simulink model "Microstick_II_33EP128MC202_Drotek_I2C_MS5611_TempAndPressure"  (Simulink 7.5)
settings: Solver=FixedStepDiscrete  StartTime=0.0  StopTime=10.0  FixedStep=0.01  RelTol=1e-3
undefined symbols (not defined in the file or in its folder): A0, A4, B10, B11, B8, B9, magnitude, Max, ms, P20, P42, P43, Pin, Resol, Slope1, Slope2, us
libraries: simulink x30, MCHP_Blockset x16
(part 2 of 2)

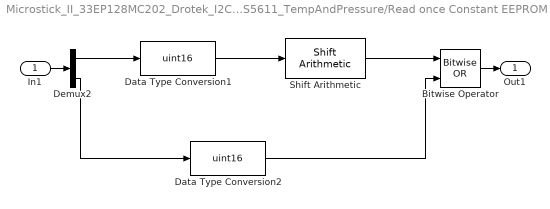
== system Microstick_II_33EP128MC202_Drotek_I2C_MS5611_TempAndPressure/Read once Constant EEPROM Calibration data From MS5611 (Blocking I2C blocks)/  ==
  In1 : Inport
  Bitwise Operator : simulink/Logic and Bit Operations/Bitwise Operator  logicop=OR  UseBitMask=off  NumInputPorts=2  BitMask=bin2dec('11011001')  BitMaskRealWorld=Stored Integer
  Data Type Conversion1 : DataTypeConversion  OutDataTypeMode=uint16  OutDataTypeStr=uint16
  Data Type Conversion2 : DataTypeConversion  OutDataTypeMode=uint16  OutDataTypeStr=uint16
  Demux2 : Demux  Outputs=2
  Shift Arithmetic : simulink/Logic and Bit Operations/Shift Arithmetic  SystemSampleTime=-1  nBitShiftRight=-8  nBinPtShiftRight=0
  Out1 : Outport
  wires:
  In1/1 -> Demux2/1
  Bitwise Operator/1 -> Out1/1
  Data Type Conversion1/1 -> Shift Arithmetic/1
  Demux2/2 -> Data Type Conversion2/1
  Shift Arithmetic/1 -> Bitwise Operator/1
  Demux2/1 -> Data Type Conversion1/1
  Data Type Conversion2/1 -> Bitwise Operator/2

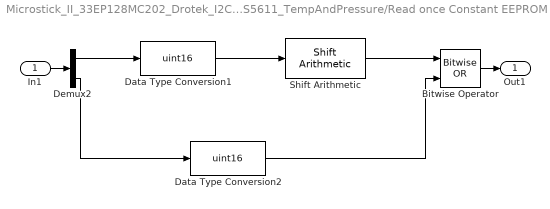
== system Microstick_II_33EP128MC202_Drotek_I2C_MS5611_TempAndPressure/Read once Constant EEPROM Calibration data From MS5611 (Blocking I2C blocks)/ 1 ==
  In1 : Inport
  Bitwise Operator : simulink/Logic and Bit Operations/Bitwise Operator  logicop=OR  UseBitMask=off  NumInputPorts=2  BitMask=bin2dec('11011001')  BitMaskRealWorld=Stored Integer
  Data Type Conversion1 : DataTypeConversion  OutDataTypeMode=uint16  OutDataTypeStr=uint16
  Data Type Conversion2 : DataTypeConversion  OutDataTypeMode=uint16  OutDataTypeStr=uint16
  Demux2 : Demux  Outputs=2
  Shift Arithmetic : simulink/Logic and Bit Operations/Shift Arithmetic  SystemSampleTime=-1  nBitShiftRight=-8  nBinPtShiftRight=0
  Out1 : Outport
  wires:
  Data Type Conversion2/1 -> Bitwise Operator/2
  Demux2/1 -> Data Type Conversion1/1
  Shift Arithmetic/1 -> Bitwise Operator/1
  Demux2/2 -> Data Type Conversion2/1
  Data Type Conversion1/1 -> Shift Arithmetic/1
  Bitwise Operator/1 -> Out1/1
  In1/1 -> Demux2/1

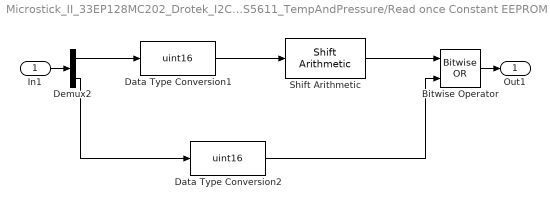
== system Microstick_II_33EP128MC202_Drotek_I2C_MS5611_TempAndPressure/Read once Constant EEPROM Calibration data From MS5611 (Blocking I2C blocks)/ 2 ==
  In1 : Inport
  Bitwise Operator : simulink/Logic and Bit Operations/Bitwise Operator  logicop=OR  UseBitMask=off  NumInputPorts=2  BitMask=bin2dec('11011001')  BitMaskRealWorld=Stored Integer
  Data Type Conversion1 : DataTypeConversion  OutDataTypeMode=uint16  OutDataTypeStr=uint16
  Data Type Conversion2 : DataTypeConversion  OutDataTypeMode=uint16  OutDataTypeStr=uint16
  Demux2 : Demux  Outputs=2
  Shift Arithmetic : simulink/Logic and Bit Operations/Shift Arithmetic  SystemSampleTime=-1  nBitShiftRight=-8  nBinPtShiftRight=0
  Out1 : Outport
  wires:
  In1/1 -> Demux2/1
  Bitwise Operator/1 -> Out1/1
  Data Type Conversion1/1 -> Shift Arithmetic/1
  Demux2/2 -> Data Type Conversion2/1
  Shift Arithmetic/1 -> Bitwise Operator/1
  Demux2/1 -> Data Type Conversion1/1
  Data Type Conversion2/1 -> Bitwise Operator/2

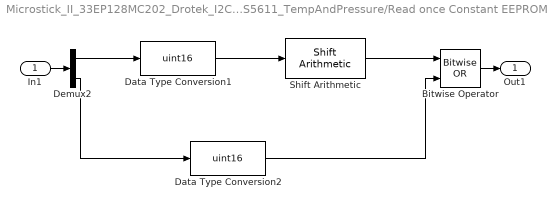
== system Microstick_II_33EP128MC202_Drotek_I2C_MS5611_TempAndPressure/Read once Constant EEPROM Calibration data From MS5611 (Blocking I2C blocks)/ 3 ==
  In1 : Inport
  Bitwise Operator : simulink/Logic and Bit Operations/Bitwise Operator  logicop=OR  UseBitMask=off  NumInputPorts=2  BitMask=bin2dec('11011001')  BitMaskRealWorld=Stored Integer
  Data Type Conversion1 : DataTypeConversion  OutDataTypeMode=uint16  OutDataTypeStr=uint16
  Data Type Conversion2 : DataTypeConversion  OutDataTypeMode=uint16  OutDataTypeStr=uint16
  Demux2 : Demux  Outputs=2
  Shift Arithmetic : simulink/Logic and Bit Operations/Shift Arithmetic  SystemSampleTime=-1  nBitShiftRight=-8  nBinPtShiftRight=0
  Out1 : Outport
  wires:
  Data Type Conversion2/1 -> Bitwise Operator/2
  Demux2/1 -> Data Type Conversion1/1
  Shift Arithmetic/1 -> Bitwise Operator/1
  Demux2/2 -> Data Type Conversion2/1
  Data Type Conversion1/1 -> Shift Arithmetic/1
  Bitwise Operator/1 -> Out1/1
  In1/1 -> Demux2/1

== system Microstick_II_33EP128MC202_Drotek_I2C_MS5611_TempAndPressure/Read once Constant EEPROM Calibration data From MS5611 (Blocking I2C blocks)/ 4 ==
  In1 : Inport
  Bitwise Operator : simulink/Logic and Bit Operations/Bitwise Operator  logicop=OR  UseBitMask=off  NumInputPorts=2  BitMask=bin2dec('11011001')  BitMaskRealWorld=Stored Integer
  Data Type Conversion1 : DataTypeConversion  OutDataTypeMode=uint16  OutDataTypeStr=uint16
  Data Type Conversion2 : DataTypeConversion  OutDataTypeMode=uint16  OutDataTypeStr=uint16
  Demux2 : Demux  Outputs=2
  Shift Arithmetic : simulink/Logic and Bit Operations/Shift Arithmetic  SystemSampleTime=-1  nBitShiftRight=-8  nBinPtShiftRight=0
  Out1 : Outport
  wires:
  In1/1 -> Demux2/1
  Bitwise Operator/1 -> Out1/1
  Data Type Conversion1/1 -> Shift Arithmetic/1
  Demux2/2 -> Data Type Conversion2/1
  Shift Arithmetic/1 -> Bitwise Operator/1
  Demux2/1 -> Data Type Conversion1/1
  Data Type Conversion2/1 -> Bitwise Operator/2

== system Microstick_II_33EP128MC202_Drotek_I2C_MS5611_TempAndPressure/Read once Constant EEPROM Calibration data From MS5611 (Blocking I2C blocks)/ 5 ==
  In1 : Inport
  Bitwise Operator : simulink/Logic and Bit Operations/Bitwise Operator  logicop=OR  UseBitMask=off  NumInputPorts=2  BitMask=bin2dec('11011001')  BitMaskRealWorld=Stored Integer
  Data Type Conversion1 : DataTypeConversion  OutDataTypeMode=uint16  OutDataTypeStr=uint16
  Data Type Conversion2 : DataTypeConversion  OutDataTypeMode=uint16  OutDataTypeStr=uint16
  Demux2 : Demux  Outputs=2
  Shift Arithmetic : simulink/Logic and Bit Operations/Shift Arithmetic  SystemSampleTime=-1  nBitShiftRight=-8  nBinPtShiftRight=0
  Out1 : Outport
  wires:
  Data Type Conversion2/1 -> Bitwise Operator/2
  Demux2/1 -> Data Type Conversion1/1
  Shift Arithmetic/1 -> Bitwise Operator/1
  Demux2/2 -> Data Type Conversion2/1
  Data Type Conversion1/1 -> Shift Arithmetic/1
  Bitwise Operator/1 -> Out1/1
  In1/1 -> Demux2/1

== system Microstick_II_33EP128MC202_Drotek_I2C_MS5611_TempAndPressure/to uint24/  ==
  In1 : Inport
  Bitwise Operator : simulink/Logic and Bit Operations/Bitwise Operator  logicop=OR  UseBitMask=off  NumInputPorts=2  BitMask=bin2dec('11011001')  BitMaskRealWorld=Stored Integer
  Data Type Conversion1 : DataTypeConversion  OutDataTypeMode=uint16  OutDataTypeStr=uint16
  Data Type Conversion2 : DataTypeConversion  OutDataTypeMode=uint16  OutDataTypeStr=uint16
  Demux2 : Demux  Outputs=2
  Shift Arithmetic : simulink/Logic and Bit Operations/Shift Arithmetic  SystemSampleTime=-1  nBitShiftRight=-8  nBinPtShiftRight=0
  Out1 : Outport
  wires:
  Data Type Conversion2/1 -> Bitwise Operator/2
  Demux2/1 -> Data Type Conversion1/1
  Shift Arithmetic/1 -> Bitwise Operator/1
  Demux2/2 -> Data Type Conversion2/1
  Data Type Conversion1/1 -> Shift Arithmetic/1
  Bitwise Operator/1 -> Out1/1
  In1/1 -> Demux2/1

== system Microstick_II_33EP128MC202_Drotek_I2C_MS5611_TempAndPressure/to uint24_/  ==
  In1 : Inport
  Bitwise Operator : simulink/Logic and Bit Operations/Bitwise Operator  logicop=OR  UseBitMask=off  NumInputPorts=2  BitMask=bin2dec('11011001')  BitMaskRealWorld=Stored Integer
  Data Type Conversion1 : DataTypeConversion  OutDataTypeMode=uint16  OutDataTypeStr=uint16
  Data Type Conversion2 : DataTypeConversion  OutDataTypeMode=uint16  OutDataTypeStr=uint16
  Demux2 : Demux  Outputs=2
  Shift Arithmetic : simulink/Logic and Bit Operations/Shift Arithmetic  SystemSampleTime=-1  nBitShiftRight=-8  nBinPtShiftRight=0
  Out1 : Outport
  wires:
  In1/1 -> Demux2/1
  Bitwise Operator/1 -> Out1/1
  Data Type Conversion1/1 -> Shift Arithmetic/1
  Demux2/2 -> Data Type Conversion2/1
  Shift Arithmetic/1 -> Bitwise Operator/1
  Demux2/1 -> Data Type Conversion1/1
  Data Type Conversion2/1 -> Bitwise Operator/2
